simulink model "PLL_3phase"  (R2022a)
settings: Solver=ode3  StartTime=0.0  StopTime=3  FixedStep=50e-6  RelTol=1e-3
InitFcn:
  | wf=2*pi*25;
libraries: spsSecondOrderFilterLib x2, spsabctodq0Lib x2, spsAlphaBetaZerotodq0Lib x1
settings Model: Creator=PSCAD_FAN  LastModifiedBy=PSCAD_FAN

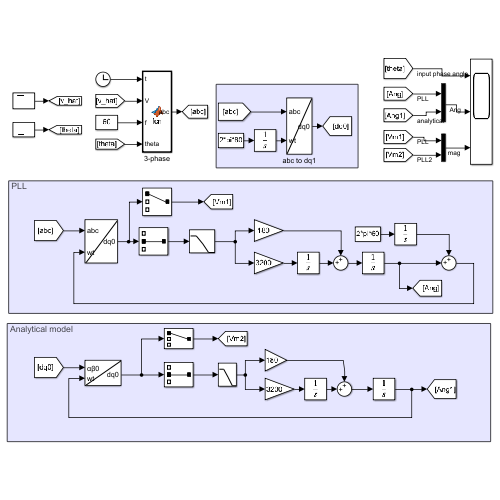
[thumbnail: Simulink's stored preview of the top-level diagram]
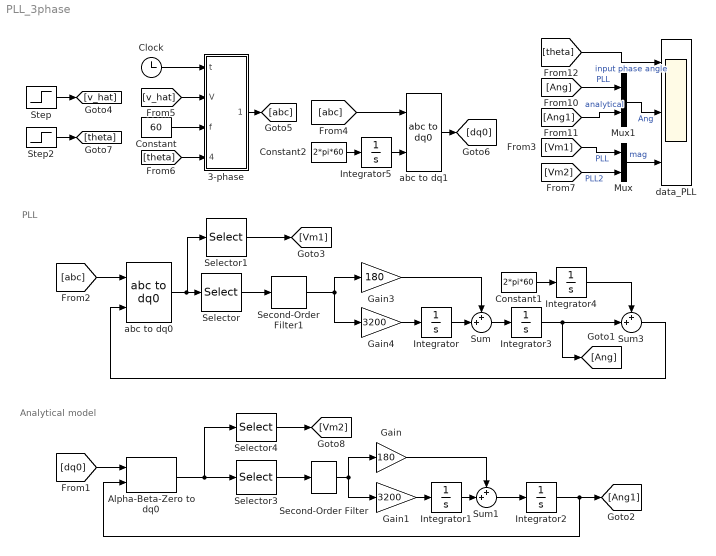
== system PLL_3phase ==
  note: Analytical model
  note: PLL
  3-phase : MATLAB Function  TreatAsAtomicUnit=on
  Alpha-Beta-Zero to dq0 : spsAlphaBetaZerotodq0Lib/Alpha-Beta-Zero to dq0  Alignment=Aligned with phase A axis
      settings: SourceProductBaseCode=PS
  Clock : Clock
  Constant : Constant  Value=60
  Constant1 : Constant  Value=2*pi*60
  Constant2 : Constant  Value=2*pi*60
  Gain : Gain  Gain=180
  Gain1 : Gain  Gain=3200
  Gain3 : Gain  Gain=180
  Gain4 : Gain  Gain=3200
  Integrator{,1..5} (6 alike) : Integrator
  Mux : Mux  Inputs=2
  Mux1 : Mux  Inputs=2
  Second-Order Filter : spsSecondOrderFilterLib/Second-Order Filter  FilterType=Lowpass  Fo=wf  Zeta=0.707  Ts=0  Initialize=on  Vac_Init="[0,  0,  60]"  Vdc_Init=0  PlotResponse=off  FreqRange=[0, 500, 1]
      settings: SourceProductBaseCode=PS
  Second-Order Filter1 : spsSecondOrderFilterLib/Second-Order Filter  FilterType=Lowpass  Fo=wf  Zeta=0.707  Ts=0  Initialize=on  Vac_Init="[0,  0,  60]"  Vdc_Init=0  PlotResponse=off  FreqRange=[0, 500, 1]
      settings: SourceProductBaseCode=PS
  Selector : Selector  InputPortWidth=3  IndexOptions=Index vector (dialog)  Indices=[2]  OutputSizes=1
  Selector1 : Selector  InputPortWidth=3  IndexOptions=Index vector (dialog)  Indices=[1]  OutputSizes=1
  Selector3 : Selector  InputPortWidth=3  IndexOptions=Index vector (dialog)  Indices=[2]  OutputSizes=1
  Selector4 : Selector  InputPortWidth=3  IndexOptions=Index vector (dialog)  Indices=[1]  OutputSizes=1
  Step : Step  Time=2  Before=1  After=0.7  SampleTime=0
  Step2 : Step  After=pi/6  SampleTime=0
  Sum : Sum  Inputs=++|
  Sum1 : Sum  Inputs=++|
  Sum3 : Sum  Inputs=++|
  abc to dq0 : spsabctodq0Lib/abc to dq0  Alignment=Aligned with phase A axis
  abc to dq1 : spsabctodq0Lib/abc to dq0  Alignment=Aligned with phase A axis
  data_PLL : Scope  NumInputPorts=3
  wires:
  Clock/1 -> 3-phase/1(t)
  Step/1 -> [v_hat]
  Constant/1 -> 3-phase/3(f)
  Step2/1 -> [theta]
  Integrator3/1 -> [Ang], Sum3/2
  [theta] -> data_PLL/1  "input phase angle"
  Second-Order Filter/1 -> Gain/1, Gain1/1
  Integrator1/1 -> Sum1/2
  Integrator2/1 -> Alpha-Beta-Zero to dq0/2, [Ang1]
  Sum1/1 -> Integrator2/1
  Gain1/1 -> Integrator1/1
  Gain/1 -> Sum1/1
  Selector3/1 -> Second-Order Filter/1
  Second-Order Filter1/1 -> Gain4/1, Gain3/1
  Sum3/1 -> abc to dq0/2
  Constant1/1 -> Integrator4/1
  Sum/1 -> Integrator3/1
  Gain4/1 -> Integrator/1
  Gain3/1 -> Sum/1
  Integrator/1 -> Sum/2
  Integrator4/1 -> Sum3/1
  3-phase/1(abc) -> [abc]
  [abc] -> abc to dq0/1
  abc to dq0/1 -> Selector1/1, Selector/1
  Selector1/1 -> [Vm1]
  Selector/1 -> Second-Order Filter1/1
  [abc] -> abc to dq1/1
  Constant2/1 -> Integrator5/1
  Integrator5/1 -> abc to dq1/2
  [v_hat] -> 3-phase/2(V)
  [theta] -> 3-phase/4(theta)
  abc to dq1/1 -> [dq0]
  Alpha-Beta-Zero to dq0/1 -> Selector4/1, Selector3/1
  Selector4/1 -> [Vm2]
  [dq0] -> Alpha-Beta-Zero to dq0/1
  Mux/1 -> data_PLL/3  "mag"
  [Vm1] -> Mux/1  "PLL"
  [Vm2] -> Mux/2  "PLL2"
  [Ang] -> Mux1/1  "PLL"
  [Ang1] -> Mux1/2  "analytical"
  Mux1/1 -> data_PLL/2  "Ang"

== matlab function PLL_3phase/3-phase ==
  data: t input; abc output; V input; f input; theta input
function abc  = fcn(t, V, f, theta)

if(t<10)
alpha = 2*pi/3; 
va = V*cos(2*pi*f*t+theta);
vb = V*cos(2*pi*f*t+theta-alpha);
vc = V*cos(2*pi*f*t+theta+ alpha);
else
    alpha = 2*pi/3; 
va = V*cos(2*pi*f*t+theta);
vb = 0.9*V*cos(2*pi*f*t+theta-alpha);
vc = V*cos(2*pi*f*t+theta+ alpha);
end


abc = [va; vb; vc];
